simulink model "Five_Car_Platoon_CS2020"  (Simulink 8.8)
settings: Solver=ode45  StartTime=0  StopTime=120  RelTol=1e-3  EnableMultiTasking=on
libraries: Solver_SF x5
settings Model: Creator=dhall  LastModifiedBy=mkhan  ExtModeTrigMode=oneshot  ExtModeArmWhenConnect=off
settings DataIOCC: LimitDataPoints=off  SignalLoggingName=sigsOut
settings OptimizationCC: BooleanDataType=off  LocalBlockOutputs=off  InitFltsAndDblsToZero=on
settings DebuggingCC: SaveWithParameterizedLinksMsg=none  SignalResolutionControl=TryResolveAllWithWarning  MultiTaskDSMMsg=warning  MultiTaskCondExecSysMsg=none  SFExecutionAtInitializationDiag=warning
settings HardwareCC: TargetUnknown=on
settings GRTTargetCC: TargetFcnLib=ansi_tfl_tmw.mat  CompOptLevelCompliant=off
settings ConfigComp: CovSFcnEnable=off

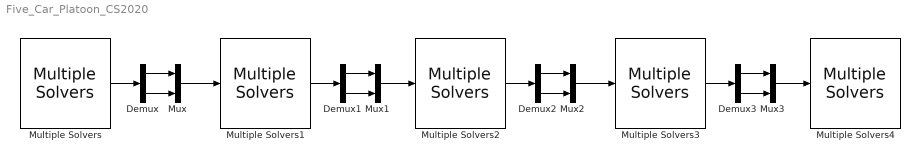
== system Five_Car_Platoon_CS2020 ==
  Demux{,1..3} (4 alike) : Demux  Outputs=2
  Multiple Solvers : Solver_SF/Multiple Solvers  Priority=1  iVehicle=1  SIMFILE=D:\mech_sim\trunk\Image\CarSim\Core\CarSim_Data\Extensions\Simulink\Multi_Vehicle\simfile1.sim  Run_RTs=off  vs_state_ind=Run  StopMode_ind=Vehicle Model  vs_scx=on
  Multiple Solvers1 : Solver_SF/Multiple Solvers  Priority=1  iVehicle=2  SIMFILE=D:\mech_sim\trunk\Image\CarSim\Core\CarSim_Data\Extensions\Simulink\Multi_Vehicle\simfile2.sim  Run_RTs=off  vs_state_ind=Run  StopMode_ind=Vehicle Model  vs_scx=on
  Multiple Solvers2 : Solver_SF/Multiple Solvers  Priority=1  iVehicle=3  SIMFILE=D:\mech_sim\trunk\Image\CarSim\Core\CarSim_Data\Extensions\Simulink\Multi_Vehicle\simfile3.sim  Run_RTs=off  vs_state_ind=Run  StopMode_ind=Vehicle Model  vs_scx=on
  Multiple Solvers3 : Solver_SF/Multiple Solvers  Priority=1  iVehicle=4  SIMFILE=D:\mech_sim\trunk\Image\CarSim\Core\CarSim_Data\Extensions\Simulink\Multi_Vehicle\simfile4.sim  Run_RTs=off  vs_state_ind=Run  StopMode_ind=Vehicle Model  vs_scx=on
  Multiple Solvers4 : Solver_SF/Multiple Solvers  Priority=1  iVehicle=5  SIMFILE=D:\mech_sim\trunk\Image\CarSim\Core\CarSim_Data\Extensions\Simulink\Multi_Vehicle\simfile5.sim  Run_RTs=off  vs_state_ind=Run  StopMode_ind=Vehicle Model  vs_scx=on
  Mux{,1..3} (4 alike) : Mux  Inputs=2
  wires:
  Multiple Solvers/1 -> Demux/1
  Demux/2 -> Mux/2
  Demux/1 -> Mux/1
  Mux/1 -> Multiple Solvers1/1
  Multiple Solvers1/1 -> Demux1/1
  Demux1/2 -> Mux1/2
  Demux1/1 -> Mux1/1
  Mux1/1 -> Multiple Solvers2/1
  Demux2/2 -> Mux2/2
  Demux2/1 -> Mux2/1
  Mux2/1 -> Multiple Solvers3/1
  Multiple Solvers3/1 -> Demux3/1
  Demux3/2 -> Mux3/2
  Demux3/1 -> Mux3/1
  Mux3/1 -> Multiple Solvers4/1
  Multiple Solvers2/1 -> Demux2/1
